simulink model "goodwin_relay"  (R2015b)
settings: Solver=ode23tb  StartTime=0.0  StopTime=tmax  RelTol=1e-3
values from neighbouring files (symbols this model uses):
  A = gamma-alpha    (= 2.5)    [added_current_fitz_relay.m]    (also in example_1.m = [0 1 1; 0 -1 6; 0 0 -1]; getAsymmetricRelayHysteresisForFitzNagumo.m = -0.5; goodwin_prediction.m = [-1 0 0 ; 1 -1 0; 0 1 -1]; new_fitz_relay.m = -1.5)
  B = 1    [added_current_fitz_relay.m]    (also in example_1.m = [1; 6; 6]; getAsymmetricRelayHysteresisForFitzNagumo.m; goodwin_prediction.m = [1; 0 ; 0]; new_fitz_relay.m)
  C = 1    [added_current_fitz_relay.m]    (also in example_1.m = [1 0 0]; getAsymmetricRelayHysteresisForFitzNagumo.m; goodwin_prediction.m = [0 0 1]; new_fitz_relay.m)
  D = 0    [added_current_fitz_relay.m]    (also in goodwin_prediction.m; new_fitz_relay.m; relay_fitz_nagumo.m; test_goodwin.m)
  X0 = a1    [added_current_fitz_relay.m]    (also in example_1.m; new_fitz_relay.m; relay_fitz_nagumo.m = a2; test_goodwin.m = [1;1;1])
settings Model: Creator=RAK  LastModifiedBy=rajiv
settings DataIOCC: LimitDataPoints=off  SaveFormat=Array
settings HardwareCC: ProdBitPerPointer=32  ProdLargestAtomicFloat=None  ProdIntDivRoundTo=Undefined  ProdEndianess=Unspecified  ProdWordSize=32  ProdHWDeviceType=32-bit Generic
settings GRTTargetCC: GeneratePreprocessorConditionals=Disable all
settings ConfigComp: CovModelRefEnable=Off

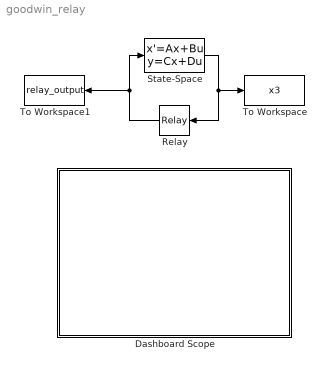
== system goodwin_relay ==
  Dashboard Scope : Subsystem  DialogController=hmiCreateDDGDialog  IsWebBlock=on  mask(MathWorksWebBlock){webBlockId=e5faaa9e-97d1-4578-9e2e-5ef7b3461644, webBlockType=sdiscope, ShowInitialText=on, HMISrcModelName=goodwin_relay}
      mask prompts: webBlockId "WebBlock Id"; webBlockType "WebBlock Type"; HMISrcModelName "Source Model"
      mask Help: helpview([docroot '/mapfiles/simulink.map'], 'hmi_scope')
      mask Display:
      | if strcmp(get_param(bdroot(gcb),'BlockDiagramType'), 'library')
      |     image([(matlabroot) '/toolbox/simulink/hmi/icons/DashboardScope.png']);
      | end
  Relay : Relay  OnSwitchValue=1  OffSwitchValue=1  OnOutputValue=0  OffOutputValue=1
  State-Space : StateSpace  A=A  B=B  C=C  D=D  X0=X0
  To Workspace : ToWorkspace  VariableName=x3  SaveFormat=Timeseries  SampleTime=-1
  To Workspace1 : ToWorkspace  VariableName=relay_output  SaveFormat=Timeseries  SampleTime=-1
  wires:
  State-Space/1 -> Relay/1, To Workspace/1
  Relay/1 -> To Workspace1/1, State-Space/1

== system goodwin_relay/Dashboard Scope ==
